simulink model "DEtest"  (R2022a)
settings: Solver=VariableStepAuto  StartTime=0.0  StopTime=10.0  RelTol=1e-3
settings Model: Creator=skundu  LastModifiedBy=skundu

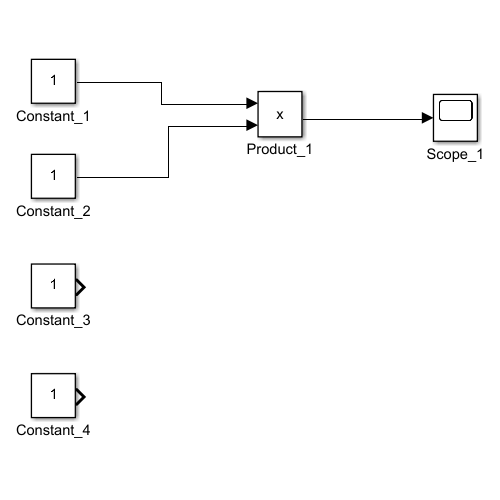
[thumbnail: Simulink's stored preview of the top-level diagram]
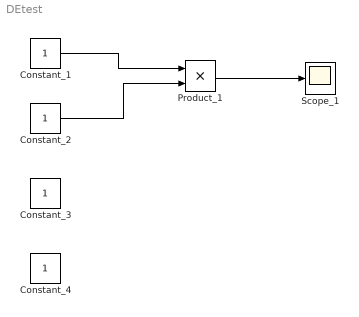
== system DEtest ==
  Constant_{1..4} (4 alike) : Constant
  Product_1 : Product
  Scope_1 : Scope
  wires:
  Constant_1/1 -> Product_1/1
  Constant_2/1 -> Product_1/2
  Product_1/1 -> Scope_1/1
